simulink model "ASL_artificial"  (R2019b)
settings: Solver=FixedStepAuto  StartTime=0.0  StopTime=10.0  FixedStep=fixedStepSize  RelTol=1e-3
undefined symbols (not defined in the file): artificial_AOT_ASL_constant, artificial_ASL_ADA_constant, ASL_resetCounterMax, ASL_subsystem1_gear, ASL_subsystem1_notAlwaysHorizon, ASL_subsystem1_speedThreshold, ASL_subsystem2_gear, ASL_subsystem2_gear2, ASL_subsystem2_notAlwaysHorizon, ASL_subsystem2_TorqueValue, ASL_subsystem2_upThreshold1, ASL_subsystem2_upThreshold2, fixedStepSize
libraries: simulink x2
settings Model: Creator=JEDDELAN  LastModifiedBy=JEDDELAN
settings DataIOCC: SaveOutput=off  SaveTime=off  ReturnWorkspaceOutputs=off
settings DebuggingCC: ArithmeticOperatorsInVariantConditions=warning
settings SFSimCC: SimUseLocalCustomCode=off  CustomCodeUndefinedFunction=UseInterfaceOnly
settings RTWCC: RTWUseLocalCustomCode=off
settings GRTTargetCC: CombineOutputUpdateFcns=off  MatFileLogging=off

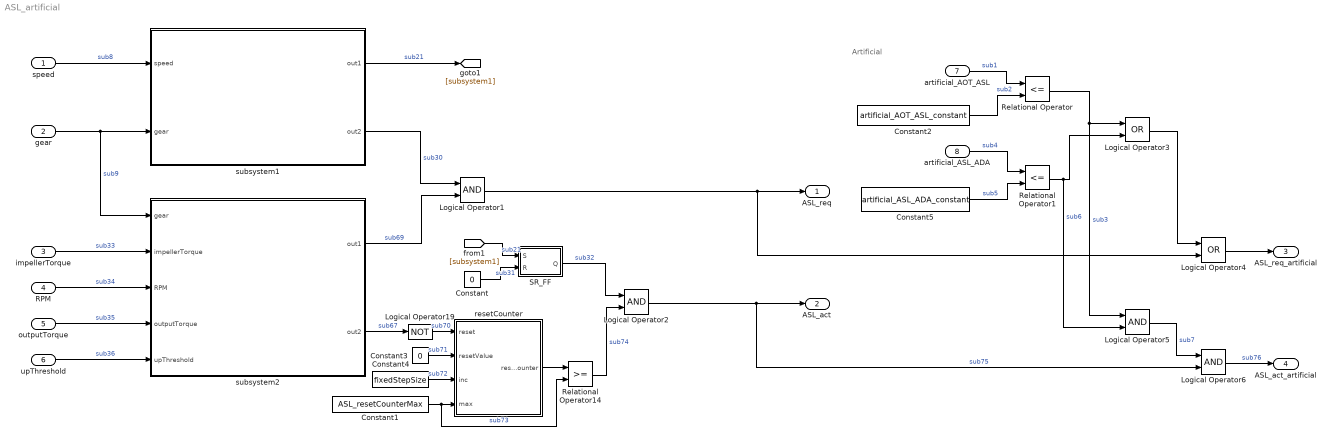
== system ASL_artificial ==
  note: Artificial
  speed : Inport
  gear : Inport  Port=2
  impellerTorque : Inport  Port=3
  RPM : Inport  Port=4
  outputTorque : Inport  Port=5
  upThreshold : Inport  Port=6
  artificial_AOT_ASL : Inport  Port=7
  artificial_ASL_ADA : Inport  Port=8
  Constant : Constant  Value=0  OutDataTypeStr=boolean
  Constant1 : Constant  Value=ASL_resetCounterMax
  Constant2 : Constant  Value=artificial_AOT_ASL_constant
  Constant3 : Constant  Value=0
  Constant4 : Constant  Value=fixedStepSize
  Constant5 : Constant  Value=artificial_ASL_ADA_constant
  Logical Operator{1..2,5..6} (4 alike) : Logic  AllPortsSameDT=off  OutDataTypeStr=boolean
  Logical Operator19 : Logic  Operator=NOT  AllPortsSameDT=off  OutDataTypeStr=boolean
  Logical Operator3 : Logic  Operator=OR  AllPortsSameDT=off  OutDataTypeStr=boolean
  Logical Operator4 : Logic  Operator=OR  AllPortsSameDT=off  OutDataTypeStr=boolean
  Relational Operator : RelationalOperator  Operator=<=  OutDataTypeStr=boolean  RndMeth=Simplest
  Relational Operator1 : RelationalOperator  Operator=<=  OutDataTypeStr=boolean  RndMeth=Simplest
  Relational Operator14 : RelationalOperator  OutDataTypeStr=boolean  RndMeth=Nearest
  SR_FF : Subsystem
      settings: CopyFcn=set_param(gcbh,'LinkStatus','none');
  resetCounter : Subsystem
      settings: CopyFcn=set_param(gcbh,'LinkStatus','none');
  subsystem1 : Subsystem
  subsystem2 : Subsystem
  ASL_req : Outport  OutDataTypeStr=boolean  PortDimensions=1  VectorParamsAs1DForOutWhenUnconnected=off
  ASL_act : Outport  Port=2  OutDataTypeStr=boolean  PortDimensions=1  VectorParamsAs1DForOutWhenUnconnected=off
  ASL_req_artificial : Outport  Port=3  OutDataTypeStr=boolean  PortDimensions=1  VectorParamsAs1DForOutWhenUnconnected=off
  ASL_act_artificial : Outport  Port=4  OutDataTypeStr=boolean  PortDimensions=1  VectorParamsAs1DForOutWhenUnconnected=off
  wires:
  gear/1 -> subsystem2/1(gear), subsystem1/2(gear)  "sub9"
  subsystem2/1(out1) -> Logical Operator1/2  "sub69"
  RPM/1 -> subsystem2/3(RPM)  "sub34"
  impellerTorque/1 -> subsystem2/2(impellerTorque)  "sub33"
  Constant/1 -> SR_FF/2(R)  "sub31"
  subsystem2/2(out2) -> Logical Operator19/1  "sub67"
  [subsystem1] -> SR_FF/1(S)  "sub21"
  upThreshold/1 -> subsystem2/5(upThreshold)  "sub36"
  resetCounter/1(resetCounter) -> Relational Operator14/1
  Constant1/1 -> resetCounter/4(max), Relational Operator14/2  "sub73"
  Constant4/1 -> resetCounter/3(inc)  "sub72"
  Logical Operator19/1 -> resetCounter/1(reset)  "sub70"
  SR_FF/1(Q) -> Logical Operator2/1  "sub32"
  subsystem1/1(out1) -> [subsystem1]  "sub21"
  subsystem1/2(out2) -> Logical Operator1/1  "sub30"
  Constant3/1 -> resetCounter/2(resetValue)  "sub71"
  Relational Operator14/1 -> Logical Operator2/2  "sub74"
  outputTorque/1 -> subsystem2/4(outputTorque)  "sub35"
  speed/1 -> subsystem1/1(speed)  "sub8"
  Constant2/1 -> Relational Operator/2  "sub2"
  Logical Operator1/1 -> Logical Operator4/2, ASL_req/1
  Logical Operator6/1 -> ASL_act_artificial/1  "sub76"
  Logical Operator5/1 -> Logical Operator6/1  "sub7"
  Relational Operator1/1 -> Logical Operator5/2, Logical Operator3/2  "sub6"
  Constant5/1 -> Relational Operator1/2  "sub5"
  Relational Operator/1 -> Logical Operator5/1, Logical Operator3/1  "sub3"
  artificial_ASL_ADA/1 -> Relational Operator1/1  "sub4"
  Logical Operator3/1 -> Logical Operator4/1
  Logical Operator2/1 -> Logical Operator6/2, ASL_act/1  "sub75"
  Logical Operator4/1 -> ASL_req_artificial/1
  artificial_AOT_ASL/1 -> Relational Operator/1  "sub1"

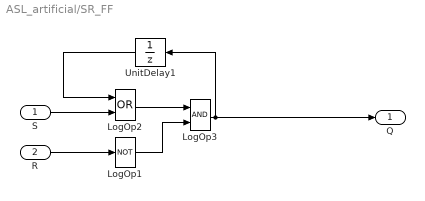
== system ASL_artificial/SR_FF ==
  S : Inport  OutDataTypeStr=boolean
  R : Inport  Port=2  OutDataTypeStr=boolean
  LogOp1 : Logic  Tag=struct('inputs','1','comment',struct('text','','placement',1),'logdata',struct('maxnumvals',4096,'plotchannels',[],'loggingmode',3,'channels',1),'operator','NOT','output',struct('class','default','description','','address','','unit','-','name','$S_$B','variable','','type','Bool'),'date',733638.68643228011,'scalingvalid',0)  Operator=NOT  Inputs=1  OutDataTypeStr=boolean
  LogOp2 : Logic  Tag=struct('inputs','2','comment',struct('text','','placement',1),'logdata',struct('maxnumvals',4096,'plotchannels',[],'loggingmode',3,'channels',1),'operator','AND','output',struct('class','default','description','','address','','unit','-','name','$S_$B','variable','','type','Bool'),'date',733638.68643680552,'scalingvalid',0)  Operator=OR  OutDataTypeStr=boolean
  LogOp3 : Logic  Tag=struct('inputs','2','comment',struct('text','','placement',1),'logdata',struct('maxnumvals',4096,'plotchannels',[],'loggingmode',3,'channels',1),'operator','OR','output',struct('class','default','description','','address','','unit','-','name','$S_$B','variable','','type','Bool'),'date',733638.68644151615,'scalingvalid',0)  OutDataTypeStr=boolean
  UnitDelay1 : UnitDelay  Tag=struct('comment',struct('text','','placement',1),'logdata',struct('maxnumvals',4096,'plotchannels',[],'loggingmode',3,'channels',1),'output',struct('width',1,'name','$S_$B','unit','','type','Bool','offset',0,'max',NaN,'min',NaN,'freeze',1,'lsb',1,'arb',0,'class','default','address','','description','','autoscalingmode',1,'lowerheadroom',1,'upperheadroom',1,'headroomunit','bit','checkmin',0,'checkmax',0,'show',0,'variable','','scaling','','keepdatatype',1,'castoutput',0),'state',struct('variable','','description','','name','X_$S_$B','width',1,'address','','max',NaN,'min',NaN,'class','default','type','Bool','scaling','','lsb',1,'offset',0,'arb',0,'freeze',1,'unit','','initial','0'),'dt','-1','date',733638.68644640048,'scalingvalid',0)  SampleTime=-1  HasFrameUpgradeWarning=on
  Q : Outport  OutDataTypeStr=boolean  VectorParamsAs1DForOutWhenUnconnected=off
  wires:
  UnitDelay1/1 -> LogOp2/1
  S/1 -> LogOp2/2
  R/1 -> LogOp1/1
  LogOp2/1 -> LogOp3/1
  LogOp1/1 -> LogOp3/2
  LogOp3/1 -> UnitDelay1/1, Q/1

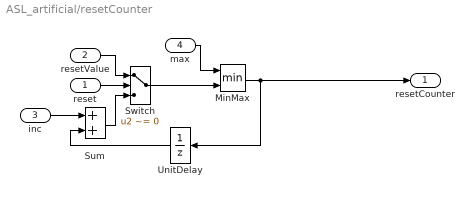
== system ASL_artificial/resetCounter ==
  reset : Inport
  resetValue : Inport  Port=2
  inc : Inport  Port=3
  max : Inport  Port=4
  MinMax : MinMax  Tag=struct('comment',struct('text','','placement',1),'inputs','2','logdata',struct('maxnumvals',4096,'plotchannels',[],'loggingmode',3,'channels',1),'output',struct('width',1,'name','$S_$B','unit','','type','Float32','offset',0,'max',NaN,'min',NaN,'freeze',1,'lsb',1,'arb',0,'class','default','address','','description','','autoscalingmode',1,'lowerheadroom',1,'upperheadroom',1,'headroomunit','bit','checkmin',0,'checkmax',0,'show',0,'variable','','scaling','','keepdatatype',1,'castoutput',0),'function','min','date',734124.44480996532,'scalingvalid',0)  Inputs=2  OutDataTypeStr=Inherit: Inherit via back propagation  InputSameDT=on
  Sum : Sum  Tag=struct('comment',struct('text','','placement',1),'logdata',struct('maxnumvals',4096,'plotchannels',[],'loggingmode',3,'channels',1),'output',struct('width',1,'name','$S_$B','unit','','type','Float32','offset',0,'max',NaN,'min',NaN,'freeze',1,'lsb',1,'arb',0,'class','default','address','','description','','autoscalingmode',1,'lowerheadroom',1,'upperheadroom',1,'headroomunit','bit','checkmin',0,'checkmax',0,'show',0,'variable','','scaling','','keepdatatype',1,'castoutput',0),'inputs','++','date',734124.44480996532,'scalingvalid',0)  OutDataTypeStr=Inherit: Same as accumulator  InputSameDT=on
  Switch : Switch  Tag=struct('comment',struct('text','','placement',1),'logdata',struct('maxnumvals',4096,'plotchannels',[],'loggingmode',3,'channels',1),'output',struct('width',1,'name','$S_$B','unit','','type','Float32','offset',0,'max',NaN,'min',NaN,'freeze',1,'lsb',1,'arb',0,'class','default','address','','description','','autoscalingmode',1,'lowerheadroom',1,'upperheadroom',1,'headroomunit','bit','checkmin',0,'checkmax',0,'show',0,'variable','','scaling','','keepdatatype',1,'castoutput',0),'threshold',struct('width',1,'name','$S_$B_threshold','unit','','type','Int16','offset',0,'max',NaN,'min',NaN,'freeze',1,'lsb',1,'arb',0,'class','default','address','','description','','value','0.5','scalar',0,'variable','','scaling','','keepdatatype',1,'criteria',1),'date',734124.4448101389,'scalingvalid',0)  Criteria=u2 ~= 0  Threshold=0.5  InputSameDT=on
  UnitDelay : UnitDelay  Tag=struct('comment',struct('text','','placement',1),'logdata',struct('maxnumvals',4096,'plotchannels',[],'loggingmode',3,'channels',1),'output',struct('width',1,'name','$S_$B','unit','','type','Float32','offset',0,'max',NaN,'min',NaN,'freeze',1,'lsb',1,'arb',0,'class','default','address','','description','','autoscalingmode',1,'lowerheadroom',1,'upperheadroom',1,'headroomunit','bit','checkmin',0,'checkmax',0,'show',0,'variable','','scaling','','keepdatatype',1,'castoutput',0),'state',struct('variable','','description','','name','X_$S_$B','width',1,'address','','max',NaN,'min',NaN,'class','default','type','Float32','scaling','','lsb',1,'offset',0,'arb',0,'freeze',1,'unit','','initial','0'),'dt','-1','date',734124.44481032412,'scalingvalid',0)  SampleTime=-1  HasFrameUpgradeWarning=on
  resetCounter : Outport  VectorParamsAs1DForOutWhenUnconnected=off
  wires:
  UnitDelay/1 -> Sum/2
  max/1 -> MinMax/1
  Switch/1 -> MinMax/2
  MinMax/1 -> UnitDelay/1, resetCounter/1
  Sum/1 -> Switch/3
  resetValue/1 -> Switch/1
  inc/1 -> Sum/1
  reset/1 -> Switch/2

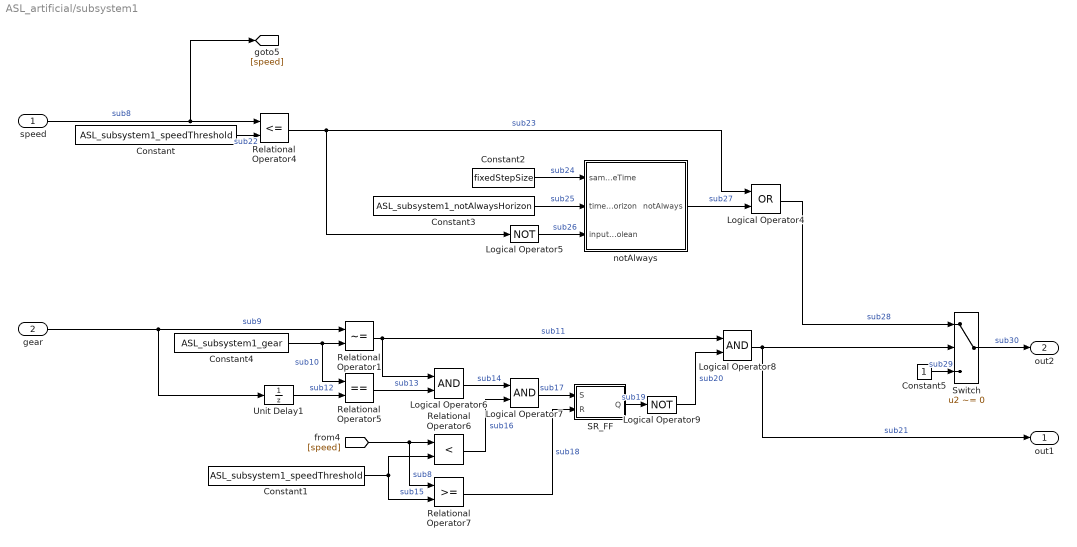
== system ASL_artificial/subsystem1 ==
  speed : Inport  Interpolate=off
  gear : Inport  Port=2
  Constant : Constant  Value=ASL_subsystem1_speedThreshold
  Constant1 : Constant  Value=ASL_subsystem1_speedThreshold
  Constant2 : Constant  Value=fixedStepSize
  Constant3 : Constant  Value=ASL_subsystem1_notAlwaysHorizon
  Constant4 : Constant  Value=ASL_subsystem1_gear
  Constant5 : Constant
  Logical Operator4 : Logic  Operator=OR  AllPortsSameDT=off  OutDataTypeStr=boolean
  Logical Operator5 : Logic  Operator=NOT  AllPortsSameDT=off  OutDataTypeStr=boolean
  Logical Operator6 : Logic  AllPortsSameDT=off  OutDataTypeStr=boolean
  Logical Operator7 : Logic  AllPortsSameDT=off  OutDataTypeStr=boolean
  Logical Operator8 : Logic  AllPortsSameDT=off  OutDataTypeStr=boolean
  Logical Operator9 : Logic  Operator=NOT  AllPortsSameDT=off  OutDataTypeStr=boolean
  Relational Operator1 : RelationalOperator  Operator=~=  OutDataTypeStr=boolean  RndMeth=Nearest
  Relational Operator4 : RelationalOperator  Operator=<=  OutDataTypeStr=boolean  RndMeth=Nearest
  Relational Operator5 : RelationalOperator  Operator===  OutDataTypeStr=boolean  RndMeth=Nearest
  Relational Operator6 : RelationalOperator  Operator=<  OutDataTypeStr=boolean  RndMeth=Nearest
  Relational Operator7 : RelationalOperator  OutDataTypeStr=boolean  RndMeth=Nearest
  SR_FF : Subsystem
      settings: CopyFcn=set_param(gcbh,'LinkStatus','none');
  Switch : Switch  Criteria=u2 ~= 0
  Unit Delay1 : UnitDelay  InitialCondition=1  SampleTime=-1  HasFrameUpgradeWarning=on
  notAlways : Subsystem
      settings: CopyFcn=set_param(gcbh,'LinkStatus','none');
  out1 : Outport  VectorParamsAs1DForOutWhenUnconnected=off
  out2 : Outport  Port=2  VectorParamsAs1DForOutWhenUnconnected=off
  wires:
  Logical Operator9/1 -> Logical Operator8/2  "sub20"
  SR_FF/1(Q) -> Logical Operator9/1  "sub19"
  Logical Operator8/1 -> Switch/2, out1/1  "sub21"
  Relational Operator7/1 -> SR_FF/2(R)  "sub18"
  Logical Operator7/1 -> SR_FF/1(S)  "sub17"
  Logical Operator6/1 -> Logical Operator7/1  "sub14"
  Relational Operator6/1 -> Logical Operator7/2  "sub16"
  Constant1/1 -> Relational Operator6/2, Relational Operator7/2  "sub15"
  [speed] -> Relational Operator6/1, Relational Operator7/1  "sub8"
  Unit Delay1/1 -> Relational Operator5/2  "sub12"
  Relational Operator5/1 -> Logical Operator6/2  "sub13"
  Logical Operator5/1 -> notAlways/3(inputBoolean)  "sub26"
  Relational Operator4/1 -> Logical Operator4/1, Logical Operator5/1  "sub23"
  notAlways/1(notAlways) -> Logical Operator4/2  "sub27"
  Logical Operator4/1 -> Switch/1  "sub28"
  Constant3/1 -> notAlways/2(timeHorizon)  "sub25"
  Constant2/1 -> notAlways/1(sampleTime)  "sub24"
  speed/1 -> [speed], Relational Operator4/1  "sub8"
  Switch/1 -> out2/1  "sub30"
  Constant5/1 -> Switch/3  "sub29"
  Relational Operator1/1 -> Logical Operator6/1, Logical Operator8/1  "sub11"
  Constant4/1 -> Relational Operator1/2, Relational Operator5/1  "sub10"
  gear/1 -> Relational Operator1/1, Unit Delay1/1  "sub9"
  Constant/1 -> Relational Operator4/2  "sub22"

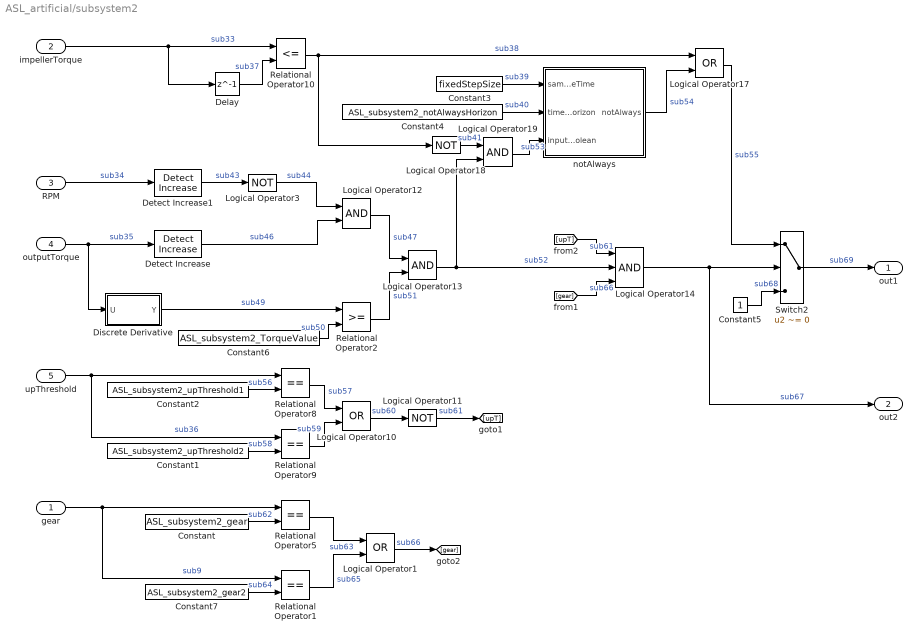
== system ASL_artificial/subsystem2 ==
  gear : Inport  Interpolate=off
  impellerTorque : Inport  Port=2
  RPM : Inport  Port=3
  outputTorque : Inport  Port=4
  upThreshold : Inport  Port=5  Interpolate=off
  Constant : Constant  Value=ASL_subsystem2_gear
  Constant1 : Constant  Value=ASL_subsystem2_upThreshold2
  Constant2 : Constant  Value=ASL_subsystem2_upThreshold1
  Constant3 : Constant  Value=fixedStepSize
  Constant4 : Constant  Value=ASL_subsystem2_notAlwaysHorizon
  Constant5 : Constant
  Constant6 : Constant  Value=ASL_subsystem2_TorqueValue
  Constant7 : Constant  Value=ASL_subsystem2_gear2
  Delay : Delay  DelayLength=1  InitialCondition=0
  Detect Increase : simulink/Logic and Bit Operations/Detect Increase  vinit=0.0  OutDataTypeStr=boolean
  Detect Increase1 : simulink/Logic and Bit Operations/Detect Increase  vinit=0.0  OutDataTypeStr=boolean
  Discrete Derivative : Subsystem
  Logical Operator1 : Logic  Operator=OR  AllPortsSameDT=off  OutDataTypeStr=boolean
  Logical Operator10 : Logic  Operator=OR  AllPortsSameDT=off  OutDataTypeStr=boolean
  Logical Operator11 : Logic  Operator=NOT  AllPortsSameDT=off  OutDataTypeStr=boolean
  Logical Operator12 : Logic  AllPortsSameDT=off  OutDataTypeStr=boolean
  Logical Operator13 : Logic  AllPortsSameDT=off  OutDataTypeStr=boolean
  Logical Operator14 : Logic  Inputs=3  AllPortsSameDT=off  OutDataTypeStr=boolean
  Logical Operator17 : Logic  Operator=OR  AllPortsSameDT=off  OutDataTypeStr=boolean
  Logical Operator18 : Logic  Operator=NOT  AllPortsSameDT=off  OutDataTypeStr=boolean
  Logical Operator19 : Logic  AllPortsSameDT=off  OutDataTypeStr=boolean
  Logical Operator3 : Logic  Operator=NOT  AllPortsSameDT=off  OutDataTypeStr=boolean
  Relational Operator{1,5,8..9} (4 alike) : RelationalOperator  Operator===  OutDataTypeStr=boolean  RndMeth=Nearest
  Relational Operator10 : RelationalOperator  Operator=<=  OutDataTypeStr=boolean  RndMeth=Nearest
  Relational Operator2 : RelationalOperator  OutDataTypeStr=boolean  RndMeth=Nearest
  Switch2 : Switch  Criteria=u2 ~= 0
  notAlways : Subsystem
      settings: CopyFcn=set_param(gcbh,'LinkStatus','none');
  out1 : Outport  VectorParamsAs1DForOutWhenUnconnected=off
  out2 : Outport  Port=2  VectorParamsAs1DForOutWhenUnconnected=off
  wires:
  Logical Operator14/1 -> Switch2/2, out2/1  "sub67"
  Relational Operator5/1 -> Logical Operator1/1  "sub63"
  Constant/1 -> Relational Operator5/2  "sub62"
  gear/1 -> Relational Operator1/1, Relational Operator5/1  "sub9"
  Logical Operator19/1 -> notAlways/3(inputBoolean)  "sub53"
  Logical Operator17/1 -> Switch2/1  "sub55"
  Constant4/1 -> notAlways/2(timeHorizon)  "sub40"
  Constant3/1 -> notAlways/1(sampleTime)  "sub39"
  Logical Operator18/1 -> Logical Operator19/1  "sub41"
  notAlways/1(notAlways) -> Logical Operator17/2  "sub54"
  Relational Operator10/1 -> Logical Operator17/1, Logical Operator18/1  "sub38"
  Delay/1 -> Relational Operator10/2  "sub37"
  impellerTorque/1 -> Relational Operator10/1, Delay/1  "sub33"
  [gear] -> Logical Operator14/3  "sub66"
  [upT] -> Logical Operator14/1  "sub61"
  Switch2/1 -> out1/1  "sub69"
  Constant5/1 -> Switch2/3  "sub68"
  Logical Operator13/1 -> Logical Operator14/2, Logical Operator19/2  "sub52"
  Discrete Derivative/1(Y) -> Relational Operator2/1  "sub49"
  Relational Operator2/1 -> Logical Operator13/2  "sub51"
  outputTorque/1 -> Discrete Derivative/1(U), Detect Increase/1  "sub35"
  Logical Operator12/1 -> Logical Operator13/1  "sub47"
  Logical Operator3/1 -> Logical Operator12/1  "sub44"
  Detect Increase/1 -> Logical Operator12/2  "sub46"
  Constant6/1 -> Relational Operator2/2  "sub50"
  Detect Increase1/1 -> Logical Operator3/1  "sub43"
  RPM/1 -> Detect Increase1/1  "sub34"
  Logical Operator11/1 -> [upT]  "sub61"
  Logical Operator10/1 -> Logical Operator11/1  "sub60"
  Relational Operator9/1 -> Logical Operator10/2  "sub59"
  Relational Operator8/1 -> Logical Operator10/1  "sub57"
  Constant1/1 -> Relational Operator9/2  "sub58"
  Constant2/1 -> Relational Operator8/2  "sub56"
  upThreshold/1 -> Relational Operator8/1, Relational Operator9/1  "sub36"
  Relational Operator1/1 -> Logical Operator1/2  "sub65"
  Constant7/1 -> Relational Operator1/2  "sub64"
  Logical Operator1/1 -> [gear]  "sub66"

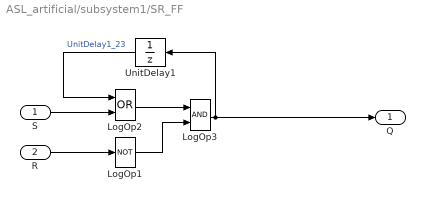
== system ASL_artificial/subsystem1/SR_FF ==
  S : Inport  OutDataTypeStr=boolean
  R : Inport  Port=2  OutDataTypeStr=boolean
  LogOp1 : Logic  Tag=struct('inputs','1','comment',struct('text','','placement',1),'logdata',struct('maxnumvals',4096,'plotchannels',[],'loggingmode',3,'channels',1),'operator','NOT','output',struct('class','default','description','','address','','unit','-','name','$S_$B','variable','','type','Bool'),'date',733638.68643228011,'scalingvalid',0)  Operator=NOT  Inputs=1  OutDataTypeStr=boolean
  LogOp2 : Logic  Tag=struct('inputs','2','comment',struct('text','','placement',1),'logdata',struct('maxnumvals',4096,'plotchannels',[],'loggingmode',3,'channels',1),'operator','AND','output',struct('class','default','description','','address','','unit','-','name','$S_$B','variable','','type','Bool'),'date',733638.68643680552,'scalingvalid',0)  Operator=OR  OutDataTypeStr=boolean
  LogOp3 : Logic  Tag=struct('inputs','2','comment',struct('text','','placement',1),'logdata',struct('maxnumvals',4096,'plotchannels',[],'loggingmode',3,'channels',1),'operator','OR','output',struct('class','default','description','','address','','unit','-','name','$S_$B','variable','','type','Bool'),'date',733638.68644151615,'scalingvalid',0)  OutDataTypeStr=boolean
  UnitDelay1 : UnitDelay  Tag=struct('comment',struct('text','','placement',1),'logdata',struct('maxnumvals',4096,'plotchannels',[],'loggingmode',3,'channels',1),'output',struct('width',1,'name','$S_$B','unit','','type','Bool','offset',0,'max',NaN,'min',NaN,'freeze',1,'lsb',1,'arb',0,'class','default','address','','description','','autoscalingmode',1,'lowerheadroom',1,'upperheadroom',1,'headroomunit','bit','checkmin',0,'checkmax',0,'show',0,'variable','','scaling','','keepdatatype',1,'castoutput',0),'state',struct('variable','','description','','name','X_$S_$B','width',1,'address','','max',NaN,'min',NaN,'class','default','type','Bool','scaling','','lsb',1,'offset',0,'arb',0,'freeze',1,'unit','','initial','0'),'dt','-1','date',733638.68644640048,'scalingvalid',0)  SampleTime=-1  HasFrameUpgradeWarning=on
  Q : Outport  OutDataTypeStr=boolean  VectorParamsAs1DForOutWhenUnconnected=off
  wires:
  UnitDelay1/1 -> LogOp2/1  "UnitDelay1_23"
  S/1 -> LogOp2/2
  R/1 -> LogOp1/1
  LogOp2/1 -> LogOp3/1
  LogOp1/1 -> LogOp3/2
  LogOp3/1 -> UnitDelay1/1, Q/1

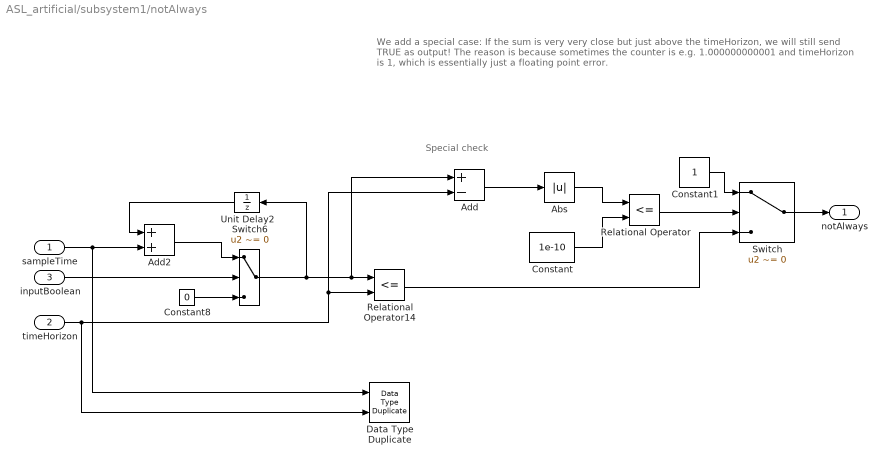
== system ASL_artificial/subsystem1/notAlways ==
  note: Special check
  note: We add a special case:
      | If the sum is very very close but just above the timeHorizon, we will still send TRUE as output!
      |
      | The reason is because sometimes the counter is e.g. 1.000000000001 and timeHorizon is 1, which is essentially just a floating point error.
  sampleTime : Inport
  timeHorizon : Inport  Port=2
  inputBoolean : Inport  Port=3
  Abs : Abs
  Add : Sum  Inputs=+-
  Add2 : Sum
  Constant : Constant  Value=1e-10
  Constant1 : Constant  OutDataTypeStr=boolean
  Constant8 : Constant  Value=0  OutDataTypeStr=Inherit: Inherit via back propagation
  Data Type Duplicate : DataTypeDuplicate
  Relational Operator : RelationalOperator  Operator=<=  OutDataTypeStr=boolean  RndMeth=Simplest
  Relational Operator14 : RelationalOperator  Operator=<=  OutDataTypeStr=boolean  RndMeth=Nearest
  Switch : Switch  Criteria=u2 ~= 0
  Switch6 : Switch  Criteria=u2 ~= 0
  Unit Delay2 : UnitDelay  SampleTime=-1  HasFrameUpgradeWarning=on
  notAlways : Outport  VectorParamsAs1DForOutWhenUnconnected=off
  wires:
  Switch6/1 -> Add/1, Relational Operator14/1, Unit Delay2/1
  timeHorizon/1 -> Add/2, Relational Operator14/2, Data Type Duplicate/2
  Relational Operator14/1 -> Switch/3
  Unit Delay2/1 -> Add2/1
  Add2/1 -> Switch6/1
  sampleTime/1 -> Add2/2, Data Type Duplicate/1
  Constant8/1 -> Switch6/3
  inputBoolean/1 -> Switch6/2
  Add/1 -> Abs/1
  Abs/1 -> Relational Operator/1
  Constant/1 -> Relational Operator/2
  Relational Operator/1 -> Switch/2
  Constant1/1 -> Switch/1
  Switch/1 -> notAlways/1

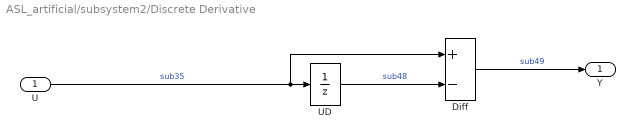
== system ASL_artificial/subsystem2/Discrete Derivative ==
  U : Inport
  Diff : Sum  Description=Add in CPU  Inputs=+-  OutMin=-10000  OutMax=100000  OutDataTypeStr=double
  UD : UnitDelay  Description=Store in Global RAM  DisableCoverage=on  SampleTime=-1  HasFrameUpgradeWarning=on
  Y : Outport  OutMin=-10000  OutMax=10000  InitialOutput=0  VectorParamsAs1DForOutWhenUnconnected=off
  wires:
  Diff/1 -> Y/1  "sub49"
  U/1 -> UD/1, Diff/1  "sub35"
  UD/1 -> Diff/2  "sub48"

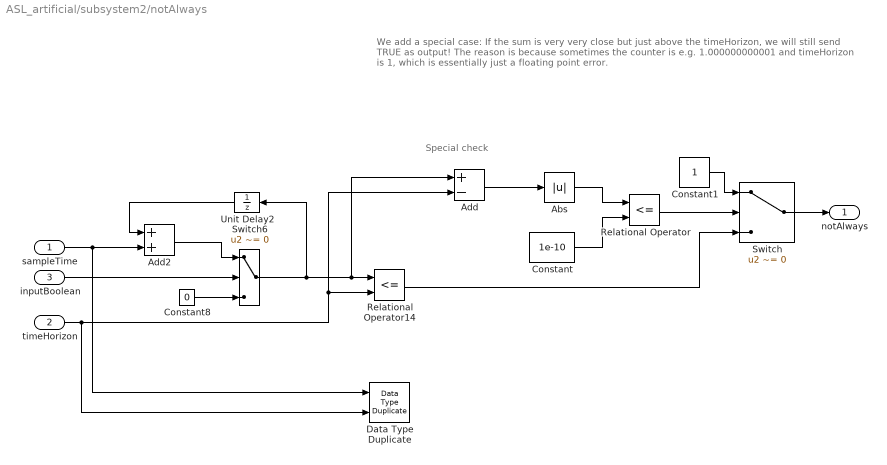
== system ASL_artificial/subsystem2/notAlways ==
  note: Special check
  note: We add a special case:
      | If the sum is very very close but just above the timeHorizon, we will still send TRUE as output!
      |
      | The reason is because sometimes the counter is e.g. 1.000000000001 and timeHorizon is 1, which is essentially just a floating point error.
  sampleTime : Inport
  timeHorizon : Inport  Port=2
  inputBoolean : Inport  Port=3
  Abs : Abs
  Add : Sum  Inputs=+-
  Add2 : Sum
  Constant : Constant  Value=1e-10
  Constant1 : Constant  OutDataTypeStr=boolean
  Constant8 : Constant  Value=0  OutDataTypeStr=Inherit: Inherit via back propagation
  Data Type Duplicate : DataTypeDuplicate
  Relational Operator : RelationalOperator  Operator=<=  OutDataTypeStr=boolean  RndMeth=Simplest
  Relational Operator14 : RelationalOperator  Operator=<=  OutDataTypeStr=boolean  RndMeth=Nearest
  Switch : Switch  Criteria=u2 ~= 0
  Switch6 : Switch  Criteria=u2 ~= 0
  Unit Delay2 : UnitDelay  SampleTime=-1  HasFrameUpgradeWarning=on
  notAlways : Outport  VectorParamsAs1DForOutWhenUnconnected=off
  wires:
  Switch6/1 -> Add/1, Relational Operator14/1, Unit Delay2/1
  timeHorizon/1 -> Add/2, Relational Operator14/2, Data Type Duplicate/2
  Relational Operator14/1 -> Switch/3
  Unit Delay2/1 -> Add2/1
  Add2/1 -> Switch6/1
  sampleTime/1 -> Add2/2, Data Type Duplicate/1
  Constant8/1 -> Switch6/3
  inputBoolean/1 -> Switch6/2
  Add/1 -> Abs/1
  Abs/1 -> Relational Operator/1
  Constant/1 -> Relational Operator/2
  Relational Operator/1 -> Switch/2
  Constant1/1 -> Switch/1
  Switch/1 -> notAlways/1
